simulink model "FourModesMerged_vrp_arp_1byte"  (R2022b)
settings: Solver=FixedStepAuto  StartTime=0.0  StopTime=10.0  FixedStep=1e-3  RelTol=1e-3  EnableMultiTasking=on
undefined symbols (not defined in the file): a, A0, A1, b, c, D0, D1, D10, D11, D12, D13, D2, D3, D4, D5, D6, D7, D8, D9, PTA0, PTA1, PTA2, PTB2, PTB23, PTB3, PTB9, PTC16, PTC17, PTC2, PTC3, PTC4, PTD0, PTD1, PTD2, PTD3
libraries: frdmk64flib x18, etargetslib x8, hdlsllib x2
settings Model: ExtModeTrigDuration=5  Creator=16475  LastModifiedBy=16475
settings OptimizationCC: EnhancedBackFolding=on  PassReuseOutputArgsAs=Individual arguments  ZeroExternalMemoryAtStartup=off  ZeroInternalMemoryAtStartup=off  MaxStackSize=64  OptimizeBlockOrder=speed  DifferentSizesBufferReuse=on  OptimizationCustomize=off  EfficientTunableParamExpr=on
settings DebuggingCC: ParameterTunabilityLossMsg=error
settings HardwareCC: ProdBitPerPointer=32  ProdBitPerSizeT=32  ProdBitPerPtrDiffT=32  ProdLargestAtomicInteger=Long  ProdLargestAtomicFloat=Double  ProdWordSize=32  ProdHWDeviceType=ARM Compatible->ARM Cortex
settings SFSimCC: MATLABDynamicMemAlloc=off
settings RTWCC: Description=Embedded Coder  SystemTargetFile=ert.tlc  HardwareBoard=NXP FRDM-K64F  TLCOptions="-aInlineSetEventsForThisBaseRateFcn=TLC_FALSE -aSuppressMultiTaskScheduler=TLC_FALSE  -aRateBasedStepFcn=0"  TemplateMakefile=ert_default_tmf  Toolchain=GNU Tools for ARM Embedded Processors
settings CodeAppCC: ForceParamTrailComments=on  IgnoreCustomStorageClasses=off  OperatorAnnotations=on  SimulinkDataObjDesc=on  SFDataObjDesc=on  InsertBlockDesc=on
settings ERTTargetCC: ExtModeTransport=4  ExtModeMexFile=sendToCommService

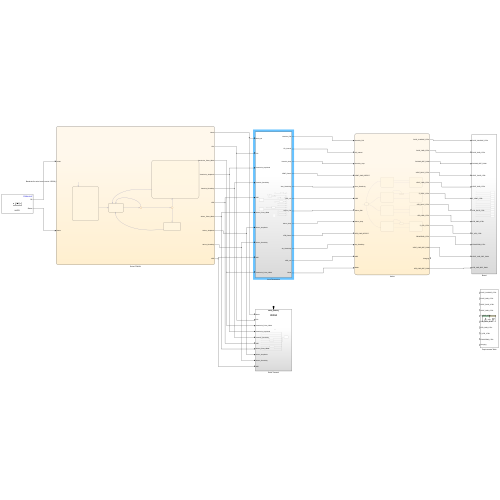
[thumbnail: Simulink's stored preview of the top-level diagram]
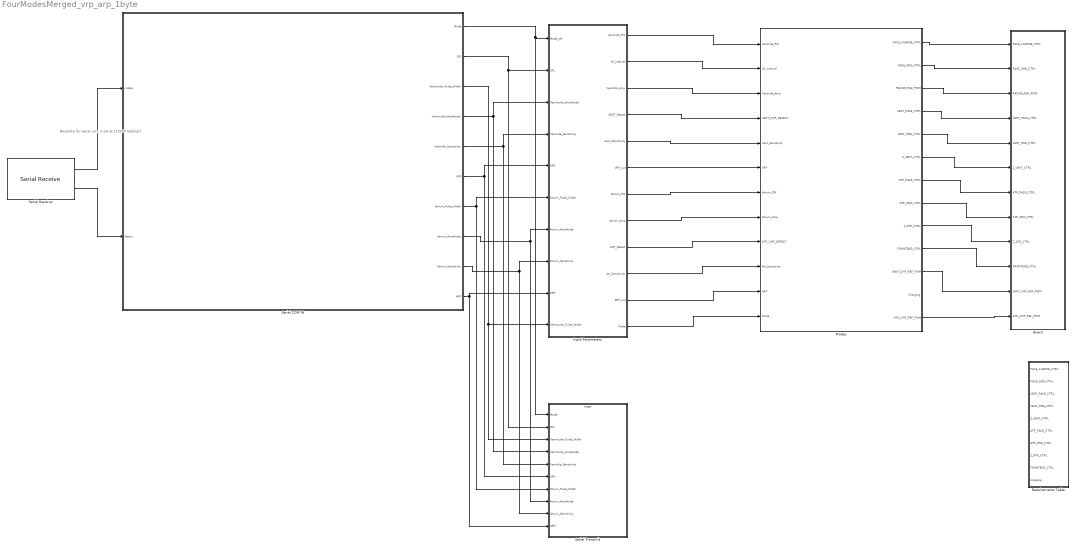
== system FourModesMerged_vrp_arp_1byte ==
  note: Baudrate for serial com is set at 115200 (default)
  Board : Subsystem
  Input Parameters : Subsystem
  Modes : Stateflow chart  TreatAsAtomicUnit=on
      settings: PortSchema="{\"entries\":[{\"content\":{\"sides\":[{\"content\":{\"connectorIds\":[\"In1\",\"In2\",\"In3\",\"In4\",\"In5\",\"In6\",\"In7\",\"In8\",\"In9\",\"In10\",\"In11\",\"In12\"]},\"type\":\"ConnectorPlacement.EquallySpacedRectSide\",\"uuid\":\"a3e94f58-3093-42a5-91db-f56c9d127bee\"},{\"content\":{\"connectorIds\":[\"Out1\",\"Out2\",\"Out3\",\"Out5\",\"Out4\",\"Out7\",\"Out6\",\"Out8\",\"Out9\",\"Out10\",\"Out11\",\"Out12\",\"Out13\"],\"side\":\"RIGHT\"},\"type\":\"ConnectorPlacement.EquallySpacedRectSide\",\"uuid\":\"289ad049-9840-4721-af22-1385d5696f7c\"},{\"content\":{\"connectorIds\":[],\"side\":\"TOP\"},\"type\":\"ConnectorPlacement.EquallySpacedRectSide\",\"uuid\":\"4602f2ad-cb91-4c7a-9db6-6571445db01f\"}]},\"type\":\"ConnectorPlacement.EquallySpacedConnector\",\"uuid\":\"bfd50937-4990-4c1b-ba87-ff4dc7d3240f\"}],\"packageUris\":[\"http://schema.mathworks.com/mf0/Connector/R2020b\"],\"version\":\"1.0\"}"
  Requirements Table : Requirements Table  TreatAsAtomicUnit=on
  Serial COM IN : Stateflow chart  TreatAsAtomicUnit=on
  Serial Receive : frdmk64flib/Serial Receive  SCIModule=0  Baudrate=uint32(9600)  Parity=None  StopBits=1  HardwareFlowControl=None  ByteOrder=LittleEndian  DataType=uint8  DataLength=26  BlockingMode=off  OutputStatus=on  SampleTime=-1
  Serial Transmit : Subsystem  TreatAsAtomicUnit=on
  wires:
  Modes/11(VENT_CMP_REF_PWM) -> Board/11(VENT_CMP_REF_PWM)
  Modes/1(PACE_CHARGE_CTRL) -> Board/1(PACE_CHARGE_CTRL)
  Modes/2(PACE_GND_CTRL) -> Board/2(PACE_GND_CTRL)
  Modes/3(PACING_REF_PWM) -> Board/3(PACING_REF_PWM)
  Modes/5(VENT_PACE_CTRL) -> Board/4(VENT_PACE_CTRL)
  Modes/4(VENT_GND_CTRL) -> Board/5(VENT_GND_CTRL)
  Modes/7(Z_VENT_CTRL) -> Board/6(Z_VENT_CTRL)
  Modes/6(ATR_PACE_CTRL) -> Board/7(ATR_PACE_CTRL)
  Modes/8(ATR_GND_CTRL) -> Board/8(ATR_GND_CTRL)
  Modes/9(Z_ATR_CTRL) -> Board/9(Z_ATR_CTRL)
  Modes/10(FRONTEND_CTRL) -> Board/10(FRONTEND_CTRL)
  Modes/13(ATR_CMP_REF_PWM) -> Board/12(ATR_CMP_REF_PWM)
  Input Parameters/1(Ventricle_PW) -> Modes/1(Ventricle_PW)
  Input Parameters/2(LR_Interval) -> Modes/2(LR_Interval)
  Input Parameters/3(Ventricle_Amp) -> Modes/3(Ventricle_Amp)
  Input Parameters/4(VENT_Detect) -> Modes/4(VENT_CMP_DETECT)
  Input Parameters/5(Vent_Sensitivity) -> Modes/5(Vent_Sensitivity)
  Input Parameters/6(VRP_out) -> Modes/6(VRP)
  Input Parameters/7(Atrium_PW) -> Modes/7(Atrium_PW)
  Input Parameters/8(Atrium_Amp) -> Modes/8(Atrium_Amp)
  Input Parameters/9(ATR_Detect) -> Modes/9(ATR_CMP_DETECT)
  Input Parameters/10(Atr_Sensitivity) -> Modes/10(Atr_Sensitivity)
  Input Parameters/11(ARP_out) -> Modes/11(ARP)
  Input Parameters/12(Mode) -> Modes/12(Mode)
  Serial Receive/1 -> Serial COM IN/1(rxdata)
  Serial Receive/2 -> Serial COM IN/2(Status)
  Serial COM IN/1(Mode) -> Serial Transmit/1(Mode), Input Parameters/1(Mode_sel)
  Serial COM IN/2(LRL) -> Serial Transmit/2(LRL), Input Parameters/2(LRL)
  Serial COM IN/3(Ventricular_Pulse_Width) -> Input Parameters/10(Ventricular_Pulse_Width), Serial Transmit/3(Ventricular_Pulse_Width)
  Serial COM IN/4(Ventricular_Amplitude) -> Serial Transmit/4(Ventricular_Amplitude), Input Parameters/3(Ventricular_Amplitude)
  Serial COM IN/5(Ventricle_Sensitivity) -> Serial Transmit/5(Ventricle_Sensitivity), Input Parameters/4(Ventricle_Sensitivity)
  Serial COM IN/6(VRP) -> Serial Transmit/6(VRP), Input Parameters/5(VRP)
  Serial COM IN/7(Atrium_Pulse_Width) -> Serial Transmit/7(Atrium_Pulse_Width), Input Parameters/6(Atrium_Pulse_Width)
  Serial COM IN/8(Atrium_Amplitude) -> Serial Transmit/8(Atrium_Amplitude), Input Parameters/7(Atrium_Amplitude)
  Serial COM IN/9(Atrium_Sensitivity) -> Serial Transmit/9(Atrium_Sensitivity), Input Parameters/8(Atrium_Sensitivity)
  Serial COM IN/10(ARP) -> Serial Transmit/10(ARP), Input Parameters/9(ARP)

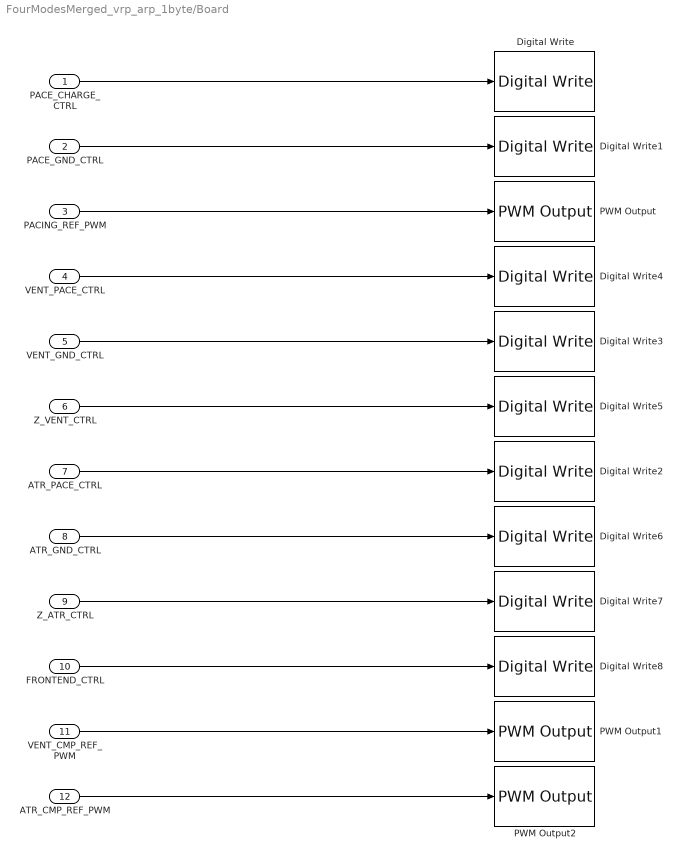
== system FourModesMerged_vrp_arp_1byte/Board ==
  PACE_CHARGE_CTRL : Inport
  PACE_GND_CTRL : Inport  Port=2
  PACING_REF_PWM : Inport  Port=3
  VENT_PACE_CTRL : Inport  Port=4
  VENT_GND_CTRL : Inport  Port=5
  Z_VENT_CTRL : Inport  Port=6
  ATR_PACE_CTRL : Inport  Port=7
  ATR_GND_CTRL : Inport  Port=8
  Z_ATR_CTRL : Inport  Port=9
  FRONTEND_CTRL : Inport  Port=10
  VENT_CMP_REF_PWM : Inport  Port=11
  ATR_CMP_REF_PWM : Inport  Port=12
  Digital Write : frdmk64flib/Digital Write  Whichpin=PTB9 (D2)
  Digital Write1 : frdmk64flib/Digital Write  Whichpin=PTD0 (D10)
  Digital Write2 : frdmk64flib/Digital Write  Whichpin=PTA0 (D8)
  Digital Write3 : frdmk64flib/Digital Write  Whichpin=PTD3 (D12)
  Digital Write4 : frdmk64flib/Digital Write  Whichpin=PTC4 (D9)
  Digital Write5 : frdmk64flib/Digital Write  Whichpin=PTC3 (D7)
  Digital Write6 : frdmk64flib/Digital Write  Whichpin=PTD2 (D11)
  Digital Write7 : frdmk64flib/Digital Write  Whichpin=PTB23 (D4)
  Digital Write8 : frdmk64flib/Digital Write  Whichpin=PTD1 (D13)
  PWM Output : frdmk64flib/PWM Output  Whichpin=PTA2 (D5)  InitialFrequency=2000  InitialDutyCycle=0
  PWM Output1 : frdmk64flib/PWM Output  Whichpin=PTA1 (D3)  InitialFrequency=2000  InitialDutyCycle=0
  PWM Output2 : frdmk64flib/PWM Output  Whichpin=PTC2 (D6)  InitialFrequency=2000  InitialDutyCycle=0
  wires:
  Z_VENT_CTRL/1 -> Digital Write5/1
  VENT_GND_CTRL/1 -> Digital Write3/1
  PACE_CHARGE_CTRL/1 -> Digital Write/1
  PACE_GND_CTRL/1 -> Digital Write1/1
  VENT_PACE_CTRL/1 -> Digital Write4/1
  ATR_GND_CTRL/1 -> Digital Write6/1
  ATR_PACE_CTRL/1 -> Digital Write2/1
  PACING_REF_PWM/1 -> PWM Output/1
  Z_ATR_CTRL/1 -> Digital Write7/1
  FRONTEND_CTRL/1 -> Digital Write8/1
  VENT_CMP_REF_PWM/1 -> PWM Output1/1
  ATR_CMP_REF_PWM/1 -> PWM Output2/1

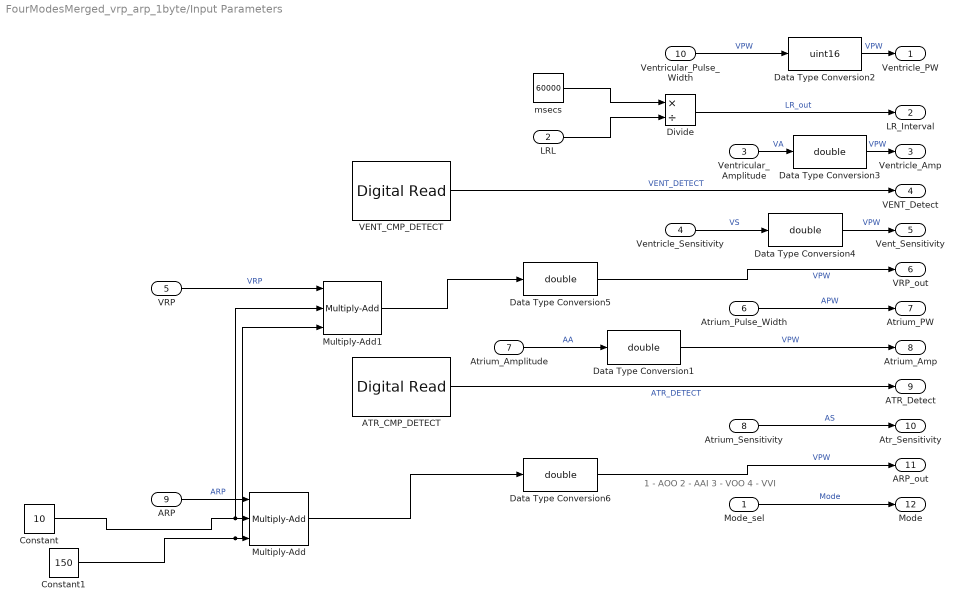
== system FourModesMerged_vrp_arp_1byte/Input Parameters ==
  note: 1 - AOO
      | 2 - AAI
      | 3 - VOO
      | 4 - VVI
  Mode_sel : Inport
  LRL : Inport  Port=2
  Ventricular_Amplitude : Inport  Port=3
  Ventricle_Sensitivity : Inport  Port=4
  VRP : Inport  Port=5  OutDataTypeStr=uint8
  Atrium_Pulse_Width : Inport  Port=6
  Atrium_Amplitude : Inport  Port=7
  Atrium_Sensitivity : Inport  Port=8
  ARP : Inport  Port=9
  Ventricular_Pulse_Width : Inport  Port=10
  ATR_CMP_DETECT : frdmk64flib/Digital Read  Whichpin=PTC16 (D0)  SampleTime=-1
  Constant : Constant  Value=10
  Constant1 : Constant  Value=150
  Data Type Conversion{1,3..6} (5 alike) : DataTypeConversion  OutDataTypeStr=double  SaturateOnIntegerOverflow=off  RndMeth=Floor
  Data Type Conversion2 : DataTypeConversion  OutDataTypeStr=uint16  SaturateOnIntegerOverflow=off  RndMeth=Floor
  Divide : Product  Inputs=*/
  Multiply-Add : hdlsllib/HDL Operations/Multiply-Add  Function=c+(a.*b)  datatype=Inherit: Inherit via internal rule  DoSatur=off  FMA=off
  Multiply-Add1 : hdlsllib/HDL Operations/Multiply-Add  Function=c+(a.*b)  datatype=Inherit: Inherit via internal rule  DoSatur=off  FMA=off
  VENT_CMP_DETECT : frdmk64flib/Digital Read  Whichpin=PTC17 (D1)  SampleTime=-1
  msecs : Constant  Value=60000
  Ventricle_PW : Outport
  LR_Interval : Outport  Port=2
  Ventricle_Amp : Outport  Port=3
  VENT_Detect : Outport  Port=4
  Vent_Sensitivity : Outport  Port=5
  VRP_out : Outport  Port=6
  Atrium_PW : Outport  Port=7
  Atrium_Amp : Outport  Port=8
  ATR_Detect : Outport  Port=9
  Atr_Sensitivity : Outport  Port=10
  ARP_out : Outport  Port=11
  Mode : Outport  Port=12
  wires:
  msecs/1 -> Divide/1
  LRL/1 -> Divide/2
  Ventricular_Pulse_Width/1 -> Data Type Conversion2/1  "VPW"
  Divide/1 -> LR_Interval/1  "LR_out"
  Ventricular_Amplitude/1 -> Data Type Conversion3/1  "VA"
  VENT_CMP_DETECT/1 -> VENT_Detect/1  "VENT_DETECT"
  Ventricle_Sensitivity/1 -> Data Type Conversion4/1  "VS"
  Atrium_Pulse_Width/1 -> Atrium_PW/1  "APW"
  Atrium_Amplitude/1 -> Data Type Conversion1/1  "AA"
  ATR_CMP_DETECT/1 -> ATR_Detect/1  "ATR_DETECT"
  Atrium_Sensitivity/1 -> Atr_Sensitivity/1  "AS"
  Mode_sel/1 -> Mode/1  "Mode"
  Data Type Conversion1/1 -> Atrium_Amp/1  "VPW"
  Data Type Conversion2/1 -> Ventricle_PW/1  "VPW"
  Data Type Conversion3/1 -> Ventricle_Amp/1  "VPW"
  Data Type Conversion4/1 -> Vent_Sensitivity/1  "VPW"
  ARP/1 -> Multiply-Add/1  "ARP"
  Constant/1 -> Multiply-Add1/2, Multiply-Add/2
  Constant1/1 -> Multiply-Add1/3, Multiply-Add/3
  Multiply-Add/1 -> Data Type Conversion6/1
  VRP/1 -> Multiply-Add1/1  "VRP"
  Multiply-Add1/1 -> Data Type Conversion5/1
  Data Type Conversion5/1 -> VRP_out/1  "VPW"
  Data Type Conversion6/1 -> ARP_out/1  "VPW"

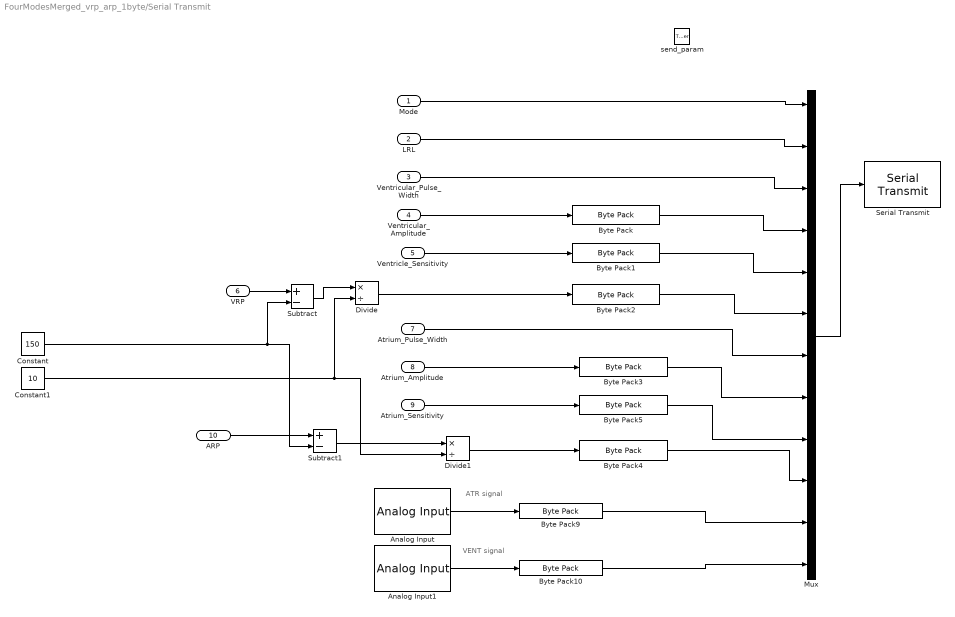
== system FourModesMerged_vrp_arp_1byte/Serial Transmit ==
  note: ATR signal
  note: VENT signal
  Mode : Inport
  LRL : Inport  Port=2
  Ventricular_Pulse_Width : Inport  Port=3
  Ventricular_Amplitude : Inport  Port=4
  Ventricle_Sensitivity : Inport  Port=5
  VRP : Inport  Port=6
  Atrium_Pulse_Width : Inport  Port=7
  Atrium_Amplitude : Inport  Port=8
  Atrium_Sensitivity : Inport  Port=9
  ARP : Inport  Port=10
  send_param : TriggerPort  TriggerType=function-call  IsSimulinkFunction=on  FunctionName=send_param  VariantControl=(inherit)
  Analog Input : frdmk64flib/Analog Input  Whichpin=PTB2 (A0)  SampleTime=-1
  Analog Input1 : frdmk64flib/Analog Input  Whichpin=PTB3 (A1)  SampleTime=-1
  Byte Pack{,1,3,5} (4 alike) : etargetslib/Byte Pack  datatypes={'single'}  byteAlign=1
  Byte Pack10 : etargetslib/Byte Pack  datatypes={'double'}  byteAlign=1
  Byte Pack2 : etargetslib/Byte Pack  datatypes={'uint8'}  byteAlign=1
  Byte Pack4 : etargetslib/Byte Pack  datatypes={'uint8'}  byteAlign=1
  Byte Pack9 : etargetslib/Byte Pack  datatypes={'double'}  byteAlign=1
  Constant : Constant  Value=150
  Constant1 : Constant  Value=10
  Divide : Product  Inputs=*/
  Divide1 : Product  Inputs=*/
  Mux : Mux  Inputs=12
  Serial Transmit : frdmk64flib/Serial Transmit  SCIModule=0  Baudrate=uint32(9600)  Parity=None  StopBits=1  HardwareFlowControl=None  ByteOrder=LittleEndian  BlockingMode=on  OutputStatus=off
  Subtract : Sum  Inputs=+-
  Subtract1 : Sum  Inputs=+-
  wires:
  Ventricular_Amplitude/1 -> Byte Pack/1
  Ventricle_Sensitivity/1 -> Byte Pack1/1
  Mux/1 -> Serial Transmit/1
  Mode/1 -> Mux/1
  LRL/1 -> Mux/2
  Ventricular_Pulse_Width/1 -> Mux/3
  Byte Pack/1 -> Mux/4
  Byte Pack1/1 -> Mux/5
  Atrium_Pulse_Width/1 -> Mux/7
  Byte Pack3/1 -> Mux/8
  Atrium_Amplitude/1 -> Byte Pack3/1
  Byte Pack5/1 -> Mux/9
  Atrium_Sensitivity/1 -> Byte Pack5/1
  Constant/1 -> Subtract1/2, Subtract/2
  VRP/1 -> Subtract/1
  ARP/1 -> Subtract1/1
  Constant1/1 -> Divide1/2, Divide/2
  Subtract/1 -> Divide/1
  Subtract1/1 -> Divide1/1
  Divide/1 -> Byte Pack2/1
  Divide1/1 -> Byte Pack4/1
  Analog Input1/1 -> Byte Pack10/1
  Analog Input/1 -> Byte Pack9/1
  Byte Pack9/1 -> Mux/11
  Byte Pack10/1 -> Mux/12
  Byte Pack2/1 -> Mux/6
  Byte Pack4/1 -> Mux/10

== stateflow chart FourModesMerged_vrp_arp_1byte/Modes ==
  state Charging_AOO
    entry:
    ATR_PACE_CTRL = false;
    VENT_PACE_CTRL = false;
    PACING_REF_PWM = ((Atrium_Amp/5)*100);
    PACE_CHARGE_CTRL = true;
    PACE_GND_CTRL = true;
    Z_ATR_CTRL = false;
    Z_VENT_CTRL = false;
    ATR_GND_CTRL = true;
    VENT_GND_CTRL = false;
    Charging = true;
  state Discharging_AOO
    entry:
    PACE_CHARGE_CTRL = false;
    PACE_GND_CTRL = true;
    ATR_PACE_CTRL = true;
    VENT_PACE_CTRL = false;
    Z_ATR_CTRL = false;
    Z_VENT_CTRL = false;
    ATR_GND_CTRL = false;
    VENT_GND_CTRL = false;
    Charging = false;
  state Charging_AAI
    entry:
    ATR_PACE_CTRL = false;
    VENT_PACE_CTRL = false;
    PACING_REF_PWM = ((Atrium_Amp/5)*100);
    PACE_CHARGE_CTRL = true;
    PACE_GND_CTRL = true;
    Z_ATR_CTRL = false;
    Z_VENT_CTRL = false;
    ATR_GND_CTRL = true;
    VENT_GND_CTRL = false;
    FRONTEND_CTRL = true;
    ATR_CMP_REF_PWM = Atr_Sensitivity;
    Charging = true;
  state Discharging_AAI
    entry:
    PACE_CHARGE_CTRL = false;
    PACE_GND_CTRL = true;
    ATR_PACE_CTRL = true;
    VENT_PACE_CTRL = false;
    Z_ATR_CTRL = false;
    Z_VENT_CTRL = false;
    ATR_GND_CTRL = false;
    VENT_GND_CTRL = false;
    FRONTEND_CTRL = false;
    Charging = false;
  state Check_State_AAI
  state Init
  state Charging_VOO
    entry:
    ATR_PACE_CTRL = false;
    VENT_PACE_CTRL = false;
    PACING_REF_PWM = ((Ventricle_Amp/5)*100);
    PACE_CHARGE_CTRL = true;
    PACE_GND_CTRL = true;
    Z_ATR_CTRL = false;
    Z_VENT_CTRL = false;
    ATR_GND_CTRL = false;
    VENT_GND_CTRL = true;
    Charging = true;
  state Discharging_VOO
    entry:
    PACE_CHARGE_CTRL = false;
    PACE_GND_CTRL = true;
    ATR_PACE_CTRL = false;
    VENT_PACE_CTRL = true;
    Z_ATR_CTRL = false;
    Z_VENT_CTRL = false;
    ATR_GND_CTRL = false;
    VENT_GND_CTRL = false;
    Charging = false;
  state Charging_Sensing_VVI
    entry:
    ATR_PACE_CTRL = false;
    VENT_PACE_CTRL = false;
    PACING_REF_PWM = ((Ventricle_Amp/5)*100);
    PACE_CHARGE_CTRL = true;
    PACE_GND_CTRL = true;
    Z_ATR_CTRL = false;
    Z_VENT_CTRL = false;
    ATR_GND_CTRL = false;
    VENT_GND_CTRL = true;
    FRONTEND_CTRL = true;
    VENT_CMP_REF_PWM = Vent_Sensitivity;
    Charging = true;
  state Discharging_VVI
    entry:
    PACE_CHARGE_CTRL = false;
    PACE_GND_CTRL = true;
    ATR_PACE_CTRL = false;
    VENT_PACE_CTRL = true;
    Z_ATR_CTRL = false;
    Z_VENT_CTRL = false;
    ATR_GND_CTRL = false;
    VENT_GND_CTRL = false;
    FRONTEND_CTRL = false;
    Charging = false;
  state Check_State_VVI
  Charging_AOO -> Discharging_AOO : [after(LR_Interval - Atrium_PW,msec)]
  Init -> Charging_AOO [order 1] : [Mode == 1]
  Discharging_AOO -> Charging_AOO : [after(Atrium_PW,msec)]
  Check_State_AAI -> Charging_AAI [order 1] : [ATR_CMP_DETECT == true]
  Charging_AAI -> Check_State_AAI : [after(ARP,msec)]
  Check_State_AAI -> Discharging_AAI [order 2] : [after(LR_Interval - ARP,msec)]
  Init -> Charging_AAI [order 2] : [Mode == 2]
  Discharging_AAI -> Charging_AAI : [after(Atrium_PW,msec)]
  (default) -> Init
  Init -> Charging_VOO [order 3] : [Mode == 3]
  Init -> Charging_Sensing_VVI [order 4] : [Mode == 4]
  Charging_VOO -> Discharging_VOO : [after(LR_Interval - Ventricle_PW,msec)]
  Discharging_VOO -> Charging_VOO : [after(Ventricle_PW,msec)]
  Check_State_VVI -> Charging_Sensing_VVI [order 1] : [VENT_CMP_DETECT == true]
  Check_State_VVI -> Discharging_VVI [order 2] : [after(LR_Interval - VRP,msec)]
  Charging_Sensing_VVI -> Check_State_VVI : [after(VRP,msec)]
  Discharging_VVI -> Charging_Sensing_VVI : [after(Ventricle_PW,msec)]
  data: Ventricle_PW input uint16; LR_Interval input double; PACE_CHARGE_CTRL output boolean; PACE_GND_CTRL output boolean; PACING_REF_PWM output double; VENT_GND_CTRL output boolean; VENT_PACE_CTRL output boolean; ATR_PACE_CTRL output boolean; Z_VENT_CTRL output boolean; Ventricle_Amp input double; ATR_GND_CTRL output boolean; Z_ATR_CTRL output boolean; VENT_CMP_DETECT input boolean; FRONTEND_CTRL output boolean; VENT_CMP_REF_PWM output double; Vent_Sensitivity input double; VRP input uint8; Charging output; Atrium_PW input; Atrium_Amp input; ATR_CMP_DETECT input; Atr_Sensitivity input; ARP input; Mode input; ATR_CMP_REF_PWM output

== stateflow chart FourModesMerged_vrp_arp_1byte/Requirements Table ==
  (default) -> (junction 1073742521)
  (junction 1073742521) -> (junction 1073742522) : {
      | % SF_REQ_REV_07
      | }
  (junction 1073742522) -> (junction 1073742524) : {
      | % HEADER_ASSIGNMENTS
      |
      | }
  (junction 1073742524) -> (junction 1073742526) : {
      | % START_A_4
      | }
  (junction 1073742526) -> (junction 1073742528) : {
      | }
  (junction 1073742528) -> (junction 1073742530)
  (junction 1073742530) -> (junction 1073742532) : {
      | }
  (junction 1073742532) -> (junction 1073742534) : {
      | % END_A_4
      | }
  (junction 1073742534) -> (junction 1073742536) : {
      | % START_R_1
      | }
  (junction 1073742536) -> (junction 1073742538) : {
      | }
  (junction 1073742538) -> (junction 1073742540)
  (junction 1073742540) -> (junction 1073742542) [order 1] : [(prev(charging) == false)]
  (junction 1073742540) -> (junction 1073742548) [order 2]
  (junction 1073742542) -> (junction 1073742544) : {
      | reqtable_postcondition((((PACE_CHARGE_CTRL) == (true))) && (((PACE_GND_CTRL) == (true))) && (((VENT_PACE_CTRL) == (false))) && (((VENT_GND_CTRL) == (true))) && (((Z_VENT_CTRL) == (false))) && (((ATR_PACE_CTRL) == (false))) && (((ATR_GND_CTRL) == (false))) && (((Z_ATR_CTRL) == (false))) && (((FRONTEND_CTRL) == (true))) && (((charging) == (true))), 'R:1');
      |
      |
      | }
  (junction 1073742544) -> (junction 1073742546) : {
      | }
  (junction 1073742546) -> (junction 1073742548)
  (junction 1073742548) -> (junction 1073742550)
  (junction 1073742550) -> (junction 1073742552) : {
      | % END_R_1
      | }
  (junction 1073742552) -> (junction 1073742554) : {
      | % START_R_7
      | }
  (junction 1073742554) -> (junction 1073742556) : {
      | }
  (junction 1073742556) -> (junction 1073742558)
  (junction 1073742558) -> (junction 1073742560) [order 1] : [(prev(charging) == true)]
  (junction 1073742558) -> (junction 1073742566) [order 2]
  (junction 1073742560) -> (junction 1073742562) : {
      | reqtable_postcondition((((PACE_CHARGE_CTRL) == (false))) && (((PACE_GND_CTRL) == (true))) && (((VENT_PACE_CTRL) == (true))) && (((VENT_GND_CTRL) == (false))) && (((Z_VENT_CTRL) == (false))) && (((ATR_PACE_CTRL) == (false))) && (((ATR_GND_CTRL) == (false))) && (((Z_ATR_CTRL) == (false))) && (((FRONTEND_CTRL) == (false))) && (((charging) == (false))), 'R:2');
      |
      |
      | }
  (junction 1073742562) -> (junction 1073742564) : {
      | }
  (junction 1073742564) -> (junction 1073742566)
  (junction 1073742566) -> (junction 1073742568)
  (junction 1073742568) -> (junction 1073742570) : {
      | % END_R_7
      | }
  data: PACE_CHARGE_CTRL input boolean; PACE_GND_CTRL input boolean; VENT_PACE_CTRL input boolean; VENT_GND_CTRL input boolean; Z_VENT_CTRL input boolean; ATR_PACE_CTRL input boolean; ATR_GND_CTRL input boolean; Z_ATR_CTRL input boolean; FRONTEND_CTRL input boolean; charging input boolean

== stateflow chart FourModesMerged_vrp_arp_1byte/Serial COM IN ==
  state SET_PARAM
    entry:
    Mode = rxdata(3);
    LRL = rxdata(4);
    Ventricular_Pulse_Width = rxdata(5);
    Ventricular_Amplitude = typecast(rxdata(6:9),'single') ;
    Ventricle_Sensitivity = typecast(rxdata(10:13),'single');
    VRP = rxdata(14);
    Atrium_Pulse_Width = rxdata(15);
    Atrium_Amplitude = typecast(rxdata(16:19),'single');
    Atrium_Sensitivity = typecast(rxdata(20:23),'single');
    ARP = rxdata(24);
  state Init
    entry:
    Mode = 1;
    Ventricular_Pulse_Width = 5;
    LRL = 120;
    Ventricular_Amplitude = 4;
    Ventricle_Sensitivity = 75;
    VRP = 150;
    Atrium_Pulse_Width = 5;
    Atrium_Amplitude = 4;
    Atrium_Sensitivity = 2.3;
    ARP = 150;
  state Standby
    %wait for COM
  state ECHO_PARAM
    entry:
    send_param();
    Egram = false;
  state Request_Egram
    entry:
    Egram = true;
    send_param();
  state Stop_Egram
    entry:
    Egram = false;
  (default) -> Init
  SET_PARAM -> Standby
  (junction 13) -> Standby [order 2]
  (junction 7) -> SET_PARAM [order 1] : [rxdata(2)==hex2dec('55')]
  Init -> Standby
  Standby -> (junction 13) [order 1] : [Status == 0]
  (junction 13) -> (junction 7) [order 1] : [rxdata(1)==hex2dec('16')]
  (junction 7) -> Stop_Egram [order 4] : [rxdata(2)==hex2dec('62')]
  (junction 7) -> Request_Egram [order 3] : [E_gram==true]
  (junction 7) -> ECHO_PARAM [order 2] : [rxdata(2)==hex2dec('22')]
  Stop_Egram -> Standby
  Standby -> Request_Egram [order 2] : [rxdata(2)==hex2dec('47')]
  Request_Egram -> Standby : after(1,msec)
  ECHO_PARAM -> Standby
  data: rxdata input uint8; Status input uint8; Mode output uint8; LRL output uint8; Ventricular_Pulse_Width output uint8; Ventricular_Amplitude output single; Ventricle_Sensitivity output single; VRP output uint8; Atrium_Pulse_Width output uint8; Atrium_Amplitude output single; Atrium_Sensitivity output single; ARP output uint8
